simulink model "Lab_6_2"  (R2016a)
settings: Solver=VariableStepAuto  StartTime=0.0  StopTime=10.0  RelTol=1e-3
settings Model: Creator=Asus  LastModifiedBy=Asus

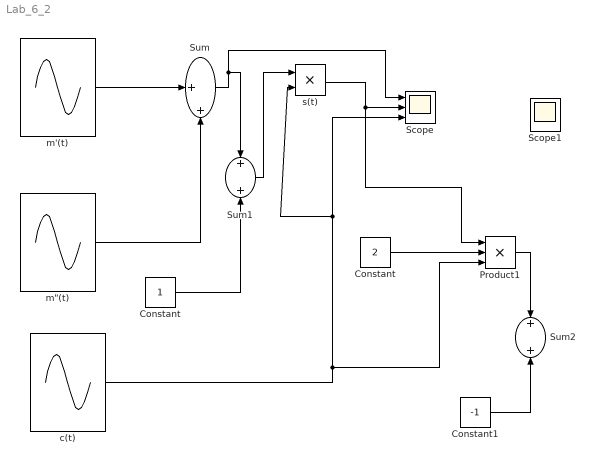
== system Lab_6_2 ==
  Constant : Constant
  "Constant " : Constant  Value=2
  Constant1 : Constant  Value=-1
  Product1 : Product  Inputs=3
  Scope : Scope  NumInputPorts=3
  Scope1 : Scope  NumInputPorts=2
  Sum : Sum  Inputs=|++
  Sum1 : Sum
  Sum2 : Sum
  c(t) : Sin  Frequency=2*pi*50  Phase=pi/2  SampleTime=1/5000
  "m\"(t)" : Sin  Amplitude=3  Frequency=2*pi*6  Phase=pi/2  SampleTime=1/5000
  m'(t) : Sin  Amplitude=2  Frequency=2*pi*4  SampleTime=1/5000
  s(t) : Product
  wires:
  m'(t)/1 -> Sum/1
  "m\"(t)"/1 -> Sum/2
  Sum1/1 -> s(t)/1
  Constant/1 -> Sum1/2
  c(t)/1 -> Product1/3, Scope/3, s(t)/2
  s(t)/1 -> Product1/1, Scope/2
  Sum/1 -> Scope/1, Sum1/1
  "Constant "/1 -> Product1/2
  Constant1/1 -> Sum2/2
  Product1/1 -> Sum2/1
